simulink model "IEEE33_SmartInverter_Physical"  (R2026a)
settings: Solver=ode23t  StopTime=2.4  MaxStep=1e-3
PreLoadFcn:
  | try, startup_project(); addpath(fullfile(pwd,'simulink_physical')); if evalin('base','exist(''simscape_pv_p_commands'',''var'')') == 0, prepare_ieee33_simscape_inputs(80,'partial_cloud','hybrid'); end; catch ME, disp(['Physical-model preload warning: ' ME.message]); end
undefined symbols (not defined in the file or in its folder): simscape_pv_capacity_kW
libraries: ee_lib x116, nesl_utility x111, fl_lib x34
(part 2 of 2)

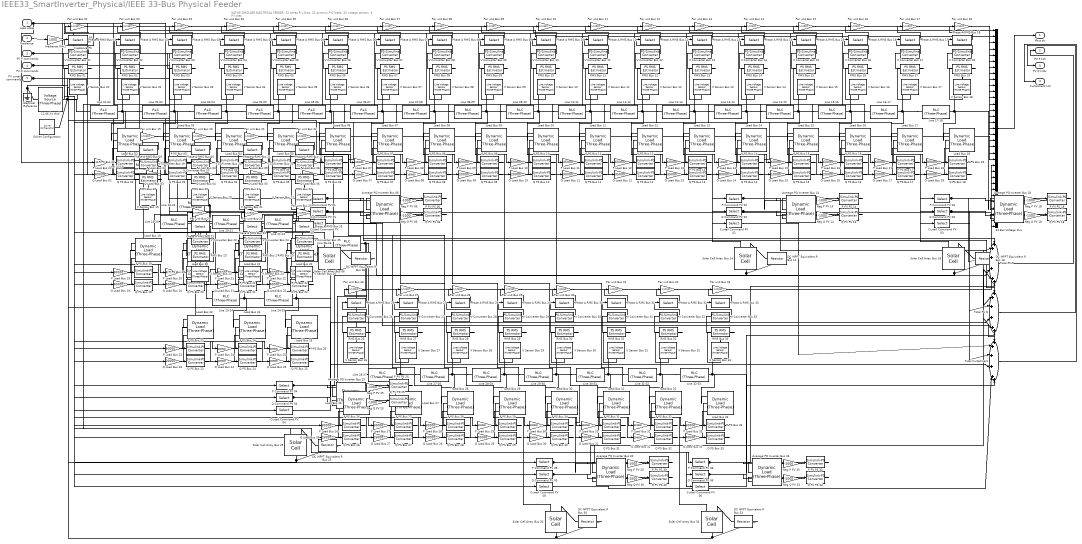
== system IEEE33_SmartInverter_Physical/IEEE 33-Bus Physical Feeder ==
  note: NATIVE SIMSCAPE ELECTRICAL FEEDER: 32 series R-L lines, 32 dynamic P-Q loads, 33 voltage sensors, 6 PV sites
  Load scale : Inport
  Irradiance : Inport  Port=2
  PV P commands : Inport  Port=3
  PV Q commands : Inport  Port=4
  PV curtail commands : Inport  Port=5
  12.66 kV Grid : ee_lib/Sources/Voltage Source (Three-Phase)  vline_rms=12660 V  shift=0 deg  freq=50 Hz  impedance_option=2  SShortCircuit=1e6 A*V  XR=15  R=0.001 Ohm  L=1e-6 H  harmonic_option=0  harmonic_orders=[5, 7, 11, 13]  harmonic_ratios=[.1, .1, .1, .1]  G_parasitic=0 1/Ohm  I_specify=off  I_priority=None  I=[0, 0, 0] A  I_nominal_specify=off  I_nominal_value=1  I_nominal_unit=A
  33 Bus Voltage Mux : Mux  Inputs=33
  Average PQ Inverter Bus 06 : ee_lib/Passive/Dynamic Load (Three-Phase)  port_option=ee.enum.threePhasePort.composite  FRated=50 Hz  Vline_rms_min=1000 V  tau=0.02 s  Vline_rms_ini=12660 V  Vang_ini=0 deg  gmin=1e-9 S
  Average PQ Inverter Bus {14,18,25,30,33} (5 alike) : ee_lib/Passive/Dynamic Load (Three-Phase)  port_option=ee.enum.threePhasePort.composite  FRated=50 Hz  Vline_rms_min=1000 V  tau=0.02 s  Vline_rms_ini=12660 V  Vang_ini=0 deg  gmin=1e-9 S
  Curtail Command PV 01 : Selector  InputPortWidth=6  IndexOptions=Index vector (dialog)  Indices=1  OutputSizes=1
  Curtail Command PV 02 : Selector  InputPortWidth=6  IndexOptions=Index vector (dialog)  Indices=2  OutputSizes=1
  Curtail Command PV 03 : Selector  InputPortWidth=6  IndexOptions=Index vector (dialog)  Indices=3  OutputSizes=1
  Curtail Command PV 04 : Selector  InputPortWidth=6  IndexOptions=Index vector (dialog)  Indices=4  OutputSizes=1
  Curtail Command PV 05 : Selector  InputPortWidth=6  IndexOptions=Index vector (dialog)  Indices=5  OutputSizes=1
  Curtail Command PV 06 : Selector  InputPortWidth=6  IndexOptions=Index vector (dialog)  Indices=6  OutputSizes=1
  DC MPPT Equivalent R Bus 06 : ee_lib/Passive/Resistor  R=(0.8*0.6*600)^2/max(simscape_pv_capacity_kW(1)*1000,1) Ohm  enable_R_tol=ee.enum.toleranceApplication.none  R_tol=5  tol_distribution=ee.enum.toleranceDistribution.uniform  nSigma=4  enable_operating_limits=ee.enum.enable.no  operating_limit_action=ee.enum.passive.reportOpLim.warn  power_rating=1 W  max_working_voltage=100 V  noise_mode=ee.enum.sources.noise.Disabled  Tdevice=25 degC  sample_time=1e-3 s  repeatability=ee.enum.ic.repeatability.notRepeatable  user_seed=0  auto_seed=3499211588  power_derating_T1=70 degC  power_derating_T2=155 degC  operating_temperature_range_vec=[-50, 150] degC  alpha=3.93e-3 1/K  Tmeas=25 degC  thermal_mass=100 J/K  temperature_specify=off  temperature_priority=High  temperature=298.15 K  temperature_nominal_specify=off  temperature_nominal_value=1  temperature_nominal_unit=K
  DC MPPT Equivalent R Bus 14 : ee_lib/Passive/Resistor  R=(0.8*0.6*600)^2/max(simscape_pv_capacity_kW(2)*1000,1) Ohm  enable_R_tol=ee.enum.toleranceApplication.none  R_tol=5  tol_distribution=ee.enum.toleranceDistribution.uniform  nSigma=4  enable_operating_limits=ee.enum.enable.no  operating_limit_action=ee.enum.passive.reportOpLim.warn  power_rating=1 W  max_working_voltage=100 V  noise_mode=ee.enum.sources.noise.Disabled  Tdevice=25 degC  sample_time=1e-3 s  repeatability=ee.enum.ic.repeatability.notRepeatable  user_seed=0  auto_seed=3890346746  power_derating_T1=70 degC  power_derating_T2=155 degC  operating_temperature_range_vec=[-50, 150] degC  alpha=3.93e-3 1/K  Tmeas=25 degC  thermal_mass=100 J/K  temperature_specify=off  temperature_priority=High  temperature=298.15 K  temperature_nominal_specify=off  temperature_nominal_value=1  temperature_nominal_unit=K
  DC MPPT Equivalent R Bus 18 : ee_lib/Passive/Resistor  R=(0.8*0.6*600)^2/max(simscape_pv_capacity_kW(3)*1000,1) Ohm  enable_R_tol=ee.enum.toleranceApplication.none  R_tol=5  tol_distribution=ee.enum.toleranceDistribution.uniform  nSigma=4  enable_operating_limits=ee.enum.enable.no  operating_limit_action=ee.enum.passive.reportOpLim.warn  power_rating=1 W  max_working_voltage=100 V  noise_mode=ee.enum.sources.noise.Disabled  Tdevice=25 degC  sample_time=1e-3 s  repeatability=ee.enum.ic.repeatability.notRepeatable  user_seed=0  auto_seed=545404223  power_derating_T1=70 degC  power_derating_T2=155 degC  operating_temperature_range_vec=[-50, 150] degC  alpha=3.93e-3 1/K  Tmeas=25 degC  thermal_mass=100 J/K  temperature_specify=off  temperature_priority=High  temperature=298.15 K  temperature_nominal_specify=off  temperature_nominal_value=1  temperature_nominal_unit=K
  DC MPPT Equivalent R Bus 25 : ee_lib/Passive/Resistor  R=(0.8*0.6*600)^2/max(simscape_pv_capacity_kW(4)*1000,1) Ohm  enable_R_tol=ee.enum.toleranceApplication.none  R_tol=5  tol_distribution=ee.enum.toleranceDistribution.uniform  nSigma=4  enable_operating_limits=ee.enum.enable.no  operating_limit_action=ee.enum.passive.reportOpLim.warn  power_rating=1 W  max_working_voltage=100 V  noise_mode=ee.enum.sources.noise.Disabled  Tdevice=25 degC  sample_time=1e-3 s  repeatability=ee.enum.ic.repeatability.notRepeatable  user_seed=0  auto_seed=3922919431  power_derating_T1=70 degC  power_derating_T2=155 degC  operating_temperature_range_vec=[-50, 150] degC  alpha=3.93e-3 1/K  Tmeas=25 degC  thermal_mass=100 J/K  temperature_specify=off  temperature_priority=High  temperature=298.15 K  temperature_nominal_specify=off  temperature_nominal_value=1  temperature_nominal_unit=K
  DC MPPT Equivalent R Bus 30 : ee_lib/Passive/Resistor  R=(0.8*0.6*600)^2/max(simscape_pv_capacity_kW(5)*1000,1) Ohm  enable_R_tol=ee.enum.toleranceApplication.none  R_tol=5  tol_distribution=ee.enum.toleranceDistribution.uniform  nSigma=4  enable_operating_limits=ee.enum.enable.no  operating_limit_action=ee.enum.passive.reportOpLim.warn  power_rating=1 W  max_working_voltage=100 V  noise_mode=ee.enum.sources.noise.Disabled  Tdevice=25 degC  sample_time=1e-3 s  repeatability=ee.enum.ic.repeatability.notRepeatable  user_seed=0  auto_seed=2715962282  power_derating_T1=70 degC  power_derating_T2=155 degC  operating_temperature_range_vec=[-50, 150] degC  alpha=3.93e-3 1/K  Tmeas=25 degC  thermal_mass=100 J/K  temperature_specify=off  temperature_priority=High  temperature=298.15 K  temperature_nominal_specify=off  temperature_nominal_value=1  temperature_nominal_unit=K
  DC MPPT Equivalent R Bus 33 : ee_lib/Passive/Resistor  R=(0.8*0.6*600)^2/max(simscape_pv_capacity_kW(6)*1000,1) Ohm  enable_R_tol=ee.enum.toleranceApplication.none  R_tol=5  tol_distribution=ee.enum.toleranceDistribution.uniform  nSigma=4  enable_operating_limits=ee.enum.enable.no  operating_limit_action=ee.enum.passive.reportOpLim.warn  power_rating=1 W  max_working_voltage=100 V  noise_mode=ee.enum.sources.noise.Disabled  Tdevice=25 degC  sample_time=1e-3 s  repeatability=ee.enum.ic.repeatability.notRepeatable  user_seed=0  auto_seed=418932850  power_derating_T1=70 degC  power_derating_T2=155 degC  operating_temperature_range_vec=[-50, 150] degC  alpha=3.93e-3 1/K  Tmeas=25 degC  thermal_mass=100 J/K  temperature_specify=off  temperature_priority=High  temperature=298.15 K  temperature_nominal_specify=off  temperature_nominal_value=1  temperature_nominal_unit=K
  Electrical Reference : fl_lib/Electrical/Electrical Elements/Electrical Reference
  Irradiance PS : nesl_utility/Simulink-PS Converter  PhysicalDomain=network_engine_domain  SubClassName=ps_input  LeftPortType=input  RightPortType=output  PseudoPeriodic=off  Frequencies=[]  NoiseDistribution=none  NoiseParameters=[]  Unit=W/m^2  AffineConversion=off  FilteringAndDerivatives=provide  SimscapeFilterOrder=1  InputFilterTimeConstant=0.001  UdotUserProvided=0
  Irradiance Wm2 : Gain  Gain=1000
  Line 01-02 : ee_lib/Passive/RLC Assemblies/RLC (Three-Phase)  port_option=ee.enum.threePhasePort.composite  component_structure=ee.enum.rlc.structure.SeriesRL  R=0.0922 Ohm  L=0.000149605646506 H  C=1e-6 F  R_parasitic=0 Ohm  G_parasitic=1e-9 1/Ohm  IL_specify=off  IL_priority=High  IL=[0, 0, 0] A  IL_nominal_specify=off  IL_nominal_value=1  IL_nominal_unit=A  VC_specify=off  VC_priority=High  VC=[0, 0, 0] V  VC_nominal_specify=off  VC_nominal_value=1  VC_nominal_unit=V
  Line 02-03 : ee_lib/Passive/RLC Assemblies/RLC (Three-Phase)  port_option=ee.enum.threePhasePort.composite  component_structure=ee.enum.rlc.structure.SeriesRL  R=0.493 Ohm  L=0.000799276124207 H  C=1e-6 F  R_parasitic=0 Ohm  G_parasitic=1e-9 1/Ohm  IL_specify=off  IL_priority=High  IL=[0, 0, 0] A  IL_nominal_specify=off  IL_nominal_value=1  IL_nominal_unit=A  VC_specify=off  VC_priority=High  VC=[0, 0, 0] V  VC_nominal_specify=off  VC_nominal_value=1  VC_nominal_unit=V
  Line 02-19 : ee_lib/Passive/RLC Assemblies/RLC (Three-Phase)  port_option=ee.enum.threePhasePort.composite  component_structure=ee.enum.rlc.structure.SeriesRL  R=0.164 Ohm  L=0.000498154971878 H  C=1e-6 F  R_parasitic=0 Ohm  G_parasitic=1e-9 1/Ohm  IL_specify=off  IL_priority=High  IL=[0, 0, 0] A  IL_nominal_specify=off  IL_nominal_value=1  IL_nominal_unit=A  VC_specify=off  VC_priority=High  VC=[0, 0, 0] V  VC_nominal_specify=off  VC_nominal_value=1  VC_nominal_unit=V
  Line 03-04 : ee_lib/Passive/RLC Assemblies/RLC (Three-Phase)  port_option=ee.enum.threePhasePort.composite  component_structure=ee.enum.rlc.structure.SeriesRL  R=0.366 Ohm  L=0.000593329627847 H  C=1e-6 F  R_parasitic=0 Ohm  G_parasitic=1e-9 1/Ohm  IL_specify=off  IL_priority=High  IL=[0, 0, 0] A  IL_nominal_specify=off  IL_nominal_value=1  IL_nominal_unit=A  VC_specify=off  VC_priority=High  VC=[0, 0, 0] V  VC_nominal_specify=off  VC_nominal_value=1  VC_nominal_unit=V
  Line 03-23 : ee_lib/Passive/RLC Assemblies/RLC (Three-Phase)  port_option=ee.enum.threePhasePort.composite  component_structure=ee.enum.rlc.structure.SeriesRL  R=0.4512 Ohm  L=0.000981349379105 H  C=1e-6 F  R_parasitic=0 Ohm  G_parasitic=1e-9 1/Ohm  IL_specify=off  IL_priority=High  IL=[0, 0, 0] A  IL_nominal_specify=off  IL_nominal_value=1  IL_nominal_unit=A  VC_specify=off  VC_priority=High  VC=[0, 0, 0] V  VC_nominal_specify=off  VC_nominal_value=1  VC_nominal_unit=V
  Line 04-05 : ee_lib/Passive/RLC Assemblies/RLC (Three-Phase)  port_option=ee.enum.threePhasePort.composite  component_structure=ee.enum.rlc.structure.SeriesRL  R=0.3811 Ohm  L=0.000617839489083 H  C=1e-6 F  R_parasitic=0 Ohm  G_parasitic=1e-9 1/Ohm  IL_specify=off  IL_priority=High  IL=[0, 0, 0] A  IL_nominal_specify=off  IL_nominal_value=1  IL_nominal_unit=A  VC_specify=off  VC_priority=High  VC=[0, 0, 0] V  VC_nominal_specify=off  VC_nominal_value=1  VC_nominal_unit=V
  Line 05-06 : ee_lib/Passive/RLC Assemblies/RLC (Three-Phase)  port_option=ee.enum.threePhasePort.composite  component_structure=ee.enum.rlc.structure.SeriesRL  R=0.819 Ohm  L=0.00225045089532 H  C=1e-6 F  R_parasitic=0 Ohm  G_parasitic=1e-9 1/Ohm  IL_specify=off  IL_priority=High  IL=[0, 0, 0] A  IL_nominal_specify=off  IL_nominal_value=1  IL_nominal_unit=A  VC_specify=off  VC_priority=High  VC=[0, 0, 0] V  VC_nominal_specify=off  VC_nominal_value=1  VC_nominal_unit=V
  Line 06-07 : ee_lib/Passive/RLC Assemblies/RLC (Three-Phase)  port_option=ee.enum.threePhasePort.composite  component_structure=ee.enum.rlc.structure.SeriesRL  R=0.1872 Ohm  L=0.00196970157571 H  C=1e-6 F  R_parasitic=0 Ohm  G_parasitic=1e-9 1/Ohm  IL_specify=off  IL_priority=High  IL=[0, 0, 0] A  IL_nominal_specify=off  IL_nominal_value=1  IL_nominal_unit=A  VC_specify=off  VC_priority=High  VC=[0, 0, 0] V  VC_nominal_specify=off  VC_nominal_value=1  VC_nominal_unit=V
  Line 06-26 : ee_lib/Passive/RLC Assemblies/RLC (Three-Phase)  port_option=ee.enum.threePhasePort.composite  component_structure=ee.enum.rlc.structure.SeriesRL  R=0.203 Ohm  L=0.000329132422314 H  C=1e-6 F  R_parasitic=0 Ohm  G_parasitic=1e-9 1/Ohm  IL_specify=off  IL_priority=High  IL=[0, 0, 0] A  IL_nominal_specify=off  IL_nominal_value=1  IL_nominal_unit=A  VC_specify=off  VC_priority=High  VC=[0, 0, 0] V  VC_nominal_specify=off  VC_nominal_value=1  VC_nominal_unit=V
  Line 07-08 : ee_lib/Passive/RLC Assemblies/RLC (Three-Phase)  port_option=ee.enum.threePhasePort.composite  component_structure=ee.enum.rlc.structure.SeriesRL  R=1.7114 Ohm  L=0.00393144540426 H  C=1e-6 F  R_parasitic=0 Ohm  G_parasitic=1e-9 1/Ohm  IL_specify=off  IL_priority=High  IL=[0, 0, 0] A  IL_nominal_specify=off  IL_nominal_value=1  IL_nominal_unit=A  VC_specify=off  VC_priority=High  VC=[0, 0, 0] V  VC_nominal_specify=off  VC_nominal_value=1  VC_nominal_unit=V
  Line 08-09 : ee_lib/Passive/RLC Assemblies/RLC (Three-Phase)  port_option=ee.enum.threePhasePort.composite  component_structure=ee.enum.rlc.structure.SeriesRL  R=1.03 Ohm  L=0.00235549315776 H  C=1e-6 F  R_parasitic=0 Ohm  G_parasitic=1e-9 1/Ohm  IL_specify=off  IL_priority=High  IL=[0, 0, 0] A  IL_nominal_specify=off  IL_nominal_value=1  IL_nominal_unit=A  VC_specify=off  VC_priority=High  VC=[0, 0, 0] V  VC_nominal_specify=off  VC_nominal_value=1  VC_nominal_unit=V
  Line 09-10 : ee_lib/Passive/RLC Assemblies/RLC (Three-Phase)  port_option=ee.enum.threePhasePort.composite  component_structure=ee.enum.rlc.structure.SeriesRL  R=1.044 Ohm  L=0.00235549315776 H  C=1e-6 F  R_parasitic=0 Ohm  G_parasitic=1e-9 1/Ohm  IL_specify=off  IL_priority=High  IL=[0, 0, 0] A  IL_nominal_specify=off  IL_nominal_value=1  IL_nominal_unit=A  VC_specify=off  VC_priority=High  VC=[0, 0, 0] V  VC_nominal_specify=off  VC_nominal_value=1  VC_nominal_unit=V
  Line 10-11 : ee_lib/Passive/RLC Assemblies/RLC (Three-Phase)  port_option=ee.enum.threePhasePort.composite  component_structure=ee.enum.rlc.structure.SeriesRL  R=0.1966 Ohm  L=0.000206901426019 H  C=1e-6 F  R_parasitic=0 Ohm  G_parasitic=1e-9 1/Ohm  IL_specify=off  IL_priority=High  IL=[0, 0, 0] A  IL_nominal_specify=off  IL_nominal_value=1  IL_nominal_unit=A  VC_specify=off  VC_priority=High  VC=[0, 0, 0] V  VC_nominal_specify=off  VC_nominal_value=1  VC_nominal_unit=V
  Line 11-12 : ee_lib/Passive/RLC Assemblies/RLC (Three-Phase)  port_option=ee.enum.threePhasePort.composite  component_structure=ee.enum.rlc.structure.SeriesRL  R=0.3744 Ohm  L=0.000394067639096 H  C=1e-6 F  R_parasitic=0 Ohm  G_parasitic=1e-9 1/Ohm  IL_specify=off  IL_priority=High  IL=[0, 0, 0] A  IL_nominal_specify=off  IL_nominal_value=1  IL_nominal_unit=A  VC_specify=off  VC_priority=High  VC=[0, 0, 0] V  VC_nominal_specify=off  VC_nominal_value=1  VC_nominal_unit=V
  Line 12-13 : ee_lib/Passive/RLC Assemblies/RLC (Three-Phase)  port_option=ee.enum.threePhasePort.composite  component_structure=ee.enum.rlc.structure.SeriesRL  R=1.468 Ohm  L=0.00367647918542 H  C=1e-6 F  R_parasitic=0 Ohm  G_parasitic=1e-9 1/Ohm  IL_specify=off  IL_priority=High  IL=[0, 0, 0] A  IL_nominal_specify=off  IL_nominal_value=1  IL_nominal_unit=A  VC_specify=off  VC_priority=High  VC=[0, 0, 0] V  VC_nominal_specify=off  VC_nominal_value=1  VC_nominal_unit=V
  Line 13-14 : ee_lib/Passive/RLC Assemblies/RLC (Three-Phase)  port_option=ee.enum.threePhasePort.composite  component_structure=ee.enum.rlc.structure.SeriesRL  R=0.5416 Ohm  L=0.0022692311786 H  C=1e-6 F  R_parasitic=0 Ohm  G_parasitic=1e-9 1/Ohm  IL_specify=off  IL_priority=High  IL=[0, 0, 0] A  IL_nominal_specify=off  IL_nominal_value=1  IL_nominal_unit=A  VC_specify=off  VC_priority=High  VC=[0, 0, 0] V  VC_nominal_specify=off  VC_nominal_value=1  VC_nominal_unit=V
  Line 14-15 : ee_lib/Passive/RLC Assemblies/RLC (Three-Phase)  port_option=ee.enum.threePhasePort.composite  component_structure=ee.enum.rlc.structure.SeriesRL  R=0.591 Ohm  L=0.00167431000133 H  C=1e-6 F  R_parasitic=0 Ohm  G_parasitic=1e-9 1/Ohm  IL_specify=off  IL_priority=High  IL=[0, 0, 0] A  IL_nominal_specify=off  IL_nominal_value=1  IL_nominal_unit=A  VC_specify=off  VC_priority=High  VC=[0, 0, 0] V  VC_nominal_specify=off  VC_nominal_value=1  VC_nominal_unit=V
  Line 15-16 : ee_lib/Passive/RLC Assemblies/RLC (Three-Phase)  port_option=ee.enum.threePhasePort.composite  component_structure=ee.enum.rlc.structure.SeriesRL  R=0.7463 Ohm  L=0.0017347888797 H  C=1e-6 F  R_parasitic=0 Ohm  G_parasitic=1e-9 1/Ohm  IL_specify=off  IL_priority=High  IL=[0, 0, 0] A  IL_nominal_specify=off  IL_nominal_value=1  IL_nominal_unit=A  VC_specify=off  VC_priority=High  VC=[0, 0, 0] V  VC_nominal_specify=off  VC_nominal_value=1  VC_nominal_unit=V
  Line 16-17 : ee_lib/Passive/RLC Assemblies/RLC (Three-Phase)  port_option=ee.enum.threePhasePort.composite  component_structure=ee.enum.rlc.structure.SeriesRL  R=1.289 Ohm  L=0.00547811314122 H  C=1e-6 F  R_parasitic=0 Ohm  G_parasitic=1e-9 1/Ohm  IL_specify=off  IL_priority=High  IL=[0, 0, 0] A  IL_nominal_specify=off  IL_nominal_value=1  IL_nominal_unit=A  VC_specify=off  VC_priority=High  VC=[0, 0, 0] V  VC_nominal_specify=off  VC_nominal_value=1  VC_nominal_unit=V
  Line 17-18 : ee_lib/Passive/RLC Assemblies/RLC (Three-Phase)  port_option=ee.enum.threePhasePort.composite  component_structure=ee.enum.rlc.structure.SeriesRL  R=0.732 Ohm  L=0.00182709874669 H  C=1e-6 F  R_parasitic=0 Ohm  G_parasitic=1e-9 1/Ohm  IL_specify=off  IL_priority=High  IL=[0, 0, 0] A  IL_nominal_specify=off  IL_nominal_value=1  IL_nominal_unit=A  VC_specify=off  VC_priority=High  VC=[0, 0, 0] V  VC_nominal_specify=off  VC_nominal_value=1  VC_nominal_unit=V
  Line 19-20 : ee_lib/Passive/RLC Assemblies/RLC (Three-Phase)  port_option=ee.enum.threePhasePort.composite  component_structure=ee.enum.rlc.structure.SeriesRL  R=1.5042 Ohm  L=0.00431437219734 H  C=1e-6 F  R_parasitic=0 Ohm  G_parasitic=1e-9 1/Ohm  IL_specify=off  IL_priority=High  IL=[0, 0, 0] A  IL_nominal_specify=off  IL_nominal_value=1  IL_nominal_unit=A  VC_specify=off  VC_priority=High  VC=[0, 0, 0] V  VC_nominal_specify=off  VC_nominal_value=1  VC_nominal_unit=V
  Line 20-21 : ee_lib/Passive/RLC Assemblies/RLC (Three-Phase)  port_option=ee.enum.threePhasePort.composite  component_structure=ee.enum.rlc.structure.SeriesRL  R=0.4095 Ohm  L=0.0015227944955 H  C=1e-6 F  R_parasitic=0 Ohm  G_parasitic=1e-9 1/Ohm  IL_specify=off  IL_priority=High  IL=[0, 0, 0] A  IL_nominal_specify=off  IL_nominal_value=1  IL_nominal_unit=A  VC_specify=off  VC_priority=High  VC=[0, 0, 0] V  VC_nominal_specify=off  VC_nominal_value=1  VC_nominal_unit=V
  Line 21-22 : ee_lib/Passive/RLC Assemblies/RLC (Three-Phase)  port_option=ee.enum.threePhasePort.composite  component_structure=ee.enum.rlc.structure.SeriesRL  R=0.7089 Ohm  L=0.0029835185632 H  C=1e-6 F  R_parasitic=0 Ohm  G_parasitic=1e-9 1/Ohm  IL_specify=off  IL_priority=High  IL=[0, 0, 0] A  IL_nominal_specify=off  IL_nominal_value=1  IL_nominal_unit=A  VC_specify=off  VC_priority=High  VC=[0, 0, 0] V  VC_nominal_specify=off  VC_nominal_value=1  VC_nominal_unit=V
  Line 23-24 : ee_lib/Passive/RLC Assemblies/RLC (Three-Phase)  port_option=ee.enum.threePhasePort.composite  component_structure=ee.enum.rlc.structure.SeriesRL  R=0.898 Ohm  L=0.00225713540293 H  C=1e-6 F  R_parasitic=0 Ohm  G_parasitic=1e-9 1/Ohm  IL_specify=off  IL_priority=High  IL=[0, 0, 0] A  IL_nominal_specify=off  IL_nominal_value=1  IL_nominal_unit=A  VC_specify=off  VC_priority=High  VC=[0, 0, 0] V  VC_nominal_specify=off  VC_nominal_value=1  VC_nominal_unit=V
  Line 24-25 : ee_lib/Passive/RLC Assemblies/RLC (Three-Phase)  port_option=ee.enum.threePhasePort.composite  component_structure=ee.enum.rlc.structure.SeriesRL  R=0.896 Ohm  L=0.00223167061203 H  C=1e-6 F  R_parasitic=0 Ohm  G_parasitic=1e-9 1/Ohm  IL_specify=off  IL_priority=High  IL=[0, 0, 0] A  IL_nominal_specify=off  IL_nominal_value=1  IL_nominal_unit=A  VC_specify=off  VC_priority=High  VC=[0, 0, 0] V  VC_nominal_specify=off  VC_nominal_value=1  VC_nominal_unit=V
  Line 26-27 : ee_lib/Passive/RLC Assemblies/RLC (Three-Phase)  port_option=ee.enum.threePhasePort.composite  component_structure=ee.enum.rlc.structure.SeriesRL  R=0.2842 Ohm  L=0.000460594405308 H  C=1e-6 F  R_parasitic=0 Ohm  G_parasitic=1e-9 1/Ohm  IL_specify=off  IL_priority=High  IL=[0, 0, 0] A  IL_nominal_specify=off  IL_nominal_value=1  IL_nominal_unit=A  VC_specify=off  VC_priority=High  VC=[0, 0, 0] V  VC_nominal_specify=off  VC_nominal_value=1  VC_nominal_unit=V
  Line 27-28 : ee_lib/Passive/RLC Assemblies/RLC (Three-Phase)  port_option=ee.enum.threePhasePort.composite  component_structure=ee.enum.rlc.structure.SeriesRL  R=1.059 Ohm  L=0.0029720594073 H  C=1e-6 F  R_parasitic=0 Ohm  G_parasitic=1e-9 1/Ohm  IL_specify=off  IL_priority=High  IL=[0, 0, 0] A  IL_nominal_specify=off  IL_nominal_value=1  IL_nominal_unit=A  VC_specify=off  VC_priority=High  VC=[0, 0, 0] V  VC_nominal_specify=off  VC_nominal_value=1  VC_nominal_unit=V
  Line 28-29 : ee_lib/Passive/RLC Assemblies/RLC (Three-Phase)  port_option=ee.enum.threePhasePort.composite  component_structure=ee.enum.rlc.structure.SeriesRL  R=0.8042 Ohm  L=0.0022300790626 H  C=1e-6 F  R_parasitic=0 Ohm  G_parasitic=1e-9 1/Ohm  IL_specify=off  IL_priority=High  IL=[0, 0, 0] A  IL_nominal_specify=off  IL_nominal_value=1  IL_nominal_unit=A  VC_specify=off  VC_priority=High  VC=[0, 0, 0] V  VC_nominal_specify=off  VC_nominal_value=1  VC_nominal_unit=V
  Line 29-30 : ee_lib/Passive/RLC Assemblies/RLC (Three-Phase)  port_option=ee.enum.threePhasePort.composite  component_structure=ee.enum.rlc.structure.SeriesRL  R=0.5075 Ohm  L=0.000822831055785 H  C=1e-6 F  R_parasitic=0 Ohm  G_parasitic=1e-9 1/Ohm  IL_specify=off  IL_priority=High  IL=[0, 0, 0] A  IL_nominal_specify=off  IL_nominal_value=1  IL_nominal_unit=A  VC_specify=off  VC_priority=High  VC=[0, 0, 0] V  VC_nominal_specify=off  VC_nominal_value=1  VC_nominal_unit=V
  Line 30-31 : ee_lib/Passive/RLC Assemblies/RLC (Three-Phase)  port_option=ee.enum.threePhasePort.composite  component_structure=ee.enum.rlc.structure.SeriesRL  R=0.9744 Ohm  L=0.00306532420395 H  C=1e-6 F  R_parasitic=0 Ohm  G_parasitic=1e-9 1/Ohm  IL_specify=off  IL_priority=High  IL=[0, 0, 0] A  IL_nominal_specify=off  IL_nominal_value=1  IL_nominal_unit=A  VC_specify=off  VC_priority=High  VC=[0, 0, 0] V  VC_nominal_specify=off  VC_nominal_value=1  VC_nominal_unit=V
  Line 31-32 : ee_lib/Passive/RLC Assemblies/RLC (Three-Phase)  port_option=ee.enum.threePhasePort.composite  component_structure=ee.enum.rlc.structure.SeriesRL  R=0.3105 Ohm  L=0.0011519634781 H  C=1e-6 F  R_parasitic=0 Ohm  G_parasitic=1e-9 1/Ohm  IL_specify=off  IL_priority=High  IL=[0, 0, 0] A  IL_nominal_specify=off  IL_nominal_value=1  IL_nominal_unit=A  VC_specify=off  VC_priority=High  VC=[0, 0, 0] V  VC_nominal_specify=off  VC_nominal_value=1  VC_nominal_unit=V
  Line 32-33 : ee_lib/Passive/RLC Assemblies/RLC (Three-Phase)  port_option=ee.enum.threePhasePort.composite  component_structure=ee.enum.rlc.structure.SeriesRL  R=0.341 Ohm  L=0.00168767901655 H  C=1e-6 F  R_parasitic=0 Ohm  G_parasitic=1e-9 1/Ohm  IL_specify=off  IL_priority=High  IL=[0, 0, 0] A  IL_nominal_specify=off  IL_nominal_value=1  IL_nominal_unit=A  VC_specify=off  VC_priority=High  VC=[0, 0, 0] V  VC_nominal_specify=off  VC_nominal_value=1  VC_nominal_unit=V
  Load Bus 02 : ee_lib/Passive/Dynamic Load (Three-Phase)  port_option=ee.enum.threePhasePort.composite  FRated=50 Hz  Vline_rms_min=1000 V  tau=0.02 s  Vline_rms_ini=12660 V  Vang_ini=0 deg  gmin=1e-9 S
  Load Bus 03 : ee_lib/Passive/Dynamic Load (Three-Phase)  port_option=ee.enum.threePhasePort.composite  FRated=50 Hz  Vline_rms_min=1000 V  tau=0.02 s  Vline_rms_ini=12660 V  Vang_ini=0 deg  gmin=1e-9 S
  Load Bus 04 : ee_lib/Passive/Dynamic Load (Three-Phase)  port_option=ee.enum.threePhasePort.composite  FRated=50 Hz  Vline_rms_min=1000 V  tau=0.02 s  Vline_rms_ini=12660 V  Vang_ini=0 deg  gmin=1e-9 S
  Load Bus 05 : ee_lib/Passive/Dynamic Load (Three-Phase)  port_option=ee.enum.threePhasePort.composite  FRated=50 Hz  Vline_rms_min=1000 V  tau=0.02 s  Vline_rms_ini=12660 V  Vang_ini=0 deg  gmin=1e-9 S
  Load Bus 06 : ee_lib/Passive/Dynamic Load (Three-Phase)  port_option=ee.enum.threePhasePort.composite  FRated=50 Hz  Vline_rms_min=1000 V  tau=0.02 s  Vline_rms_ini=12660 V  Vang_ini=0 deg  gmin=1e-9 S
  Load Bus 07 : ee_lib/Passive/Dynamic Load (Three-Phase)  port_option=ee.enum.threePhasePort.composite  FRated=50 Hz  Vline_rms_min=1000 V  tau=0.02 s  Vline_rms_ini=12660 V  Vang_ini=0 deg  gmin=1e-9 S
  Load Bus 08 : ee_lib/Passive/Dynamic Load (Three-Phase)  port_option=ee.enum.threePhasePort.composite  FRated=50 Hz  Vline_rms_min=1000 V  tau=0.02 s  Vline_rms_ini=12660 V  Vang_ini=0 deg  gmin=1e-9 S
  Load Bus 09 : ee_lib/Passive/Dynamic Load (Three-Phase)  port_option=ee.enum.threePhasePort.composite  FRated=50 Hz  Vline_rms_min=1000 V  tau=0.02 s  Vline_rms_ini=12660 V  Vang_ini=0 deg  gmin=1e-9 S
  Load Bus {10..33} (24 alike) : ee_lib/Passive/Dynamic Load (Three-Phase)  port_option=ee.enum.threePhasePort.composite  FRated=50 Hz  Vline_rms_min=1000 V  tau=0.02 s  Vline_rms_ini=12660 V  Vang_ini=0 deg  gmin=1e-9 S
  Neg P PV 06 : Gain  Gain=-1000
  Neg P PV {14,18,25,30,33} (5 alike) : Gain  Gain=-1000
  Neg Q PV 06 : Gain  Gain=-1000
  Neg Q PV {14,18,25,30,33} (5 alike) : Gain  Gain=-1000
  P Command PV 01 : Selector  InputPortWidth=6  IndexOptions=Index vector (dialog)  Indices=1  OutputSizes=1
  P Command PV 02 : Selector  InputPortWidth=6  IndexOptions=Index vector (dialog)  Indices=2  OutputSizes=1
  P Command PV 03 : Selector  InputPortWidth=6  IndexOptions=Index vector (dialog)  Indices=3  OutputSizes=1
  P Command PV 04 : Selector  InputPortWidth=6  IndexOptions=Index vector (dialog)  Indices=4  OutputSizes=1
  P Command PV 05 : Selector  InputPortWidth=6  IndexOptions=Index vector (dialog)  Indices=5  OutputSizes=1
  P Command PV 06 : Selector  InputPortWidth=6  IndexOptions=Index vector (dialog)  Indices=6  OutputSizes=1
  P Load Bus 02 : Gain  Gain=100000
  P Load Bus 03 : Gain  Gain=90000
  P Load Bus 04 : Gain  Gain=120000
  P Load Bus 05 : Gain  Gain=60000
  P Load Bus 06 : Gain  Gain=60000
  P Load Bus 07 : Gain  Gain=200000
  P Load Bus 08 : Gain  Gain=200000
  P Load Bus 09 : Gain  Gain=60000
  P Load Bus {10,12..13,15..17,26..28,33} (10 alike) : Gain  Gain=60000
  P Load Bus 11 : Gain  Gain=45000
  P Load Bus 14 : Gain  Gain=120000
  P Load Bus {18..23} (6 alike) : Gain  Gain=90000
  P Load Bus 24 : Gain  Gain=420000
  P Load Bus 25 : Gain  Gain=420000
  P Load Bus 29 : Gain  Gain=120000
  P Load Bus 30 : Gain  Gain=200000
  P Load Bus 31 : Gain  Gain=150000
  P Load Bus 32 : Gain  Gain=210000
  P PS Bus 02 : nesl_utility/Simulink-PS Converter  PhysicalDomain=network_engine_domain  SubClassName=ps_input  LeftPortType=input  RightPortType=output  PseudoPeriodic=off  Frequencies=[]  NoiseDistribution=none  NoiseParameters=[]  Unit=W  AffineConversion=off  FilteringAndDerivatives=provide  SimscapeFilterOrder=1  InputFilterTimeConstant=0.001  UdotUserProvided=0
  P PS Bus 03 : nesl_utility/Simulink-PS Converter  PhysicalDomain=network_engine_domain  SubClassName=ps_input  LeftPortType=input  RightPortType=output  PseudoPeriodic=off  Frequencies=[]  NoiseDistribution=none  NoiseParameters=[]  Unit=W  AffineConversion=off  FilteringAndDerivatives=provide  SimscapeFilterOrder=1  InputFilterTimeConstant=0.001  UdotUserProvided=0
  P PS Bus 04 : nesl_utility/Simulink-PS Converter  PhysicalDomain=network_engine_domain  SubClassName=ps_input  LeftPortType=input  RightPortType=output  PseudoPeriodic=off  Frequencies=[]  NoiseDistribution=none  NoiseParameters=[]  Unit=W  AffineConversion=off  FilteringAndDerivatives=provide  SimscapeFilterOrder=1  InputFilterTimeConstant=0.001  UdotUserProvided=0
  P PS Bus 05 : nesl_utility/Simulink-PS Converter  PhysicalDomain=network_engine_domain  SubClassName=ps_input  LeftPortType=input  RightPortType=output  PseudoPeriodic=off  Frequencies=[]  NoiseDistribution=none  NoiseParameters=[]  Unit=W  AffineConversion=off  FilteringAndDerivatives=provide  SimscapeFilterOrder=1  InputFilterTimeConstant=0.001  UdotUserProvided=0
  P PS Bus 06 : nesl_utility/Simulink-PS Converter  PhysicalDomain=network_engine_domain  SubClassName=ps_input  LeftPortType=input  RightPortType=output  PseudoPeriodic=off  Frequencies=[]  NoiseDistribution=none  NoiseParameters=[]  Unit=W  AffineConversion=off  FilteringAndDerivatives=provide  SimscapeFilterOrder=1  InputFilterTimeConstant=0.001  UdotUserProvided=0
  P PS Bus 07 : nesl_utility/Simulink-PS Converter  PhysicalDomain=network_engine_domain  SubClassName=ps_input  LeftPortType=input  RightPortType=output  PseudoPeriodic=off  Frequencies=[]  NoiseDistribution=none  NoiseParameters=[]  Unit=W  AffineConversion=off  FilteringAndDerivatives=provide  SimscapeFilterOrder=1  InputFilterTimeConstant=0.001  UdotUserProvided=0
  P PS Bus 08 : nesl_utility/Simulink-PS Converter  PhysicalDomain=network_engine_domain  SubClassName=ps_input  LeftPortType=input  RightPortType=output  PseudoPeriodic=off  Frequencies=[]  NoiseDistribution=none  NoiseParameters=[]  Unit=W  AffineConversion=off  FilteringAndDerivatives=provide  SimscapeFilterOrder=1  InputFilterTimeConstant=0.001  UdotUserProvided=0
  P PS Bus 09 : nesl_utility/Simulink-PS Converter  PhysicalDomain=network_engine_domain  SubClassName=ps_input  LeftPortType=input  RightPortType=output  PseudoPeriodic=off  Frequencies=[]  NoiseDistribution=none  NoiseParameters=[]  Unit=W  AffineConversion=off  FilteringAndDerivatives=provide  SimscapeFilterOrder=1  InputFilterTimeConstant=0.001  UdotUserProvided=0
  P PS Bus {10..33} (24 alike) : nesl_utility/Simulink-PS Converter  PhysicalDomain=network_engine_domain  SubClassName=ps_input  LeftPortType=input  RightPortType=output  PseudoPeriodic=off  Frequencies=[]  NoiseDistribution=none  NoiseParameters=[]  Unit=W  AffineConversion=off  FilteringAndDerivatives=provide  SimscapeFilterOrder=1  InputFilterTimeConstant=0.001  UdotUserProvided=0
  P PV PS 06 : nesl_utility/Simulink-PS Converter  PhysicalDomain=network_engine_domain  SubClassName=ps_input  LeftPortType=input  RightPortType=output  PseudoPeriodic=off  Frequencies=[]  NoiseDistribution=none  NoiseParameters=[]  Unit=W  AffineConversion=off  FilteringAndDerivatives=provide  SimscapeFilterOrder=1  InputFilterTimeConstant=0.001  UdotUserProvided=0
  P PV PS {14,18,25,30,33} (5 alike) : nesl_utility/Simulink-PS Converter  PhysicalDomain=network_engine_domain  SubClassName=ps_input  LeftPortType=input  RightPortType=output  PseudoPeriodic=off  Frequencies=[]  NoiseDistribution=none  NoiseParameters=[]  Unit=W  AffineConversion=off  FilteringAndDerivatives=provide  SimscapeFilterOrder=1  InputFilterTimeConstant=0.001  UdotUserProvided=0
  Per unit Bus 01 : Gain  Gain=1/12660
  Per unit Bus 02 : Gain  Gain=1/12660
  Per unit Bus 03 : Gain  Gain=1/12660
  Per unit Bus 04 : Gain  Gain=1/12660
  Per unit Bus 05 : Gain  Gain=1/12660
  Per unit Bus 06 : Gain  Gain=1/12660
  Per unit Bus 07 : Gain  Gain=1/12660
  Per unit Bus 08 : Gain  Gain=1/12660
  Per unit Bus 09 : Gain  Gain=1/12660
  Per unit Bus {10..33} (24 alike) : Gain  Gain=1/12660
  Phase A RMS Bus 01 : Selector  InputPortWidth=3  IndexOptions=Index vector (dialog)  Indices=1  OutputSizes=1
  Phase A RMS Bus 02 : Selector  InputPortWidth=3  IndexOptions=Index vector (dialog)  Indices=1  OutputSizes=1
  Phase A RMS Bus 03 : Selector  InputPortWidth=3  IndexOptions=Index vector (dialog)  Indices=1  OutputSizes=1
  Phase A RMS Bus 04 : Selector  InputPortWidth=3  IndexOptions=Index vector (dialog)  Indices=1  OutputSizes=1
  Phase A RMS Bus 05 : Selector  InputPortWidth=3  IndexOptions=Index vector (dialog)  Indices=1  OutputSizes=1
  Phase A RMS Bus 06 : Selector  InputPortWidth=3  IndexOptions=Index vector (dialog)  Indices=1  OutputSizes=1
  Phase A RMS Bus 07 : Selector  InputPortWidth=3  IndexOptions=Index vector (dialog)  Indices=1  OutputSizes=1
  Phase A RMS Bus 08 : Selector  InputPortWidth=3  IndexOptions=Index vector (dialog)  Indices=1  OutputSizes=1
  Phase A RMS Bus 09 : Selector  InputPortWidth=3  IndexOptions=Index vector (dialog)  Indices=1  OutputSizes=1
  Phase A RMS Bus {10..33} (24 alike) : Selector  InputPortWidth=3  IndexOptions=Index vector (dialog)  Indices=1  OutputSizes=1
  Q Command PV 01 : Selector  InputPortWidth=6  IndexOptions=Index vector (dialog)  Indices=1  OutputSizes=1
  Q Command PV 02 : Selector  InputPortWidth=6  IndexOptions=Index vector (dialog)  Indices=2  OutputSizes=1
  Q Command PV 03 : Selector  InputPortWidth=6  IndexOptions=Index vector (dialog)  Indices=3  OutputSizes=1
  Q Command PV 04 : Selector  InputPortWidth=6  IndexOptions=Index vector (dialog)  Indices=4  OutputSizes=1
  Q Command PV 05 : Selector  InputPortWidth=6  IndexOptions=Index vector (dialog)  Indices=5  OutputSizes=1
  Q Command PV 06 : Selector  InputPortWidth=6  IndexOptions=Index vector (dialog)  Indices=6  OutputSizes=1
  Q Load Bus 02 : Gain  Gain=60000
  Q Load Bus 03 : Gain  Gain=40000
  Q Load Bus 04 : Gain  Gain=80000
  Q Load Bus 05 : Gain  Gain=30000
  Q Load Bus 06 : Gain  Gain=20000
  Q Load Bus 07 : Gain  Gain=100000
  Q Load Bus 08 : Gain  Gain=100000
  Q Load Bus 09 : Gain  Gain=20000
  Q Load Bus {10,16..17,28} (4 alike) : Gain  Gain=20000
  Q Load Bus 11 : Gain  Gain=30000
  Q Load Bus 12 : Gain  Gain=35000
  Q Load Bus 13 : Gain  Gain=35000
  Q Load Bus 14 : Gain  Gain=80000
  Q Load Bus 15 : Gain  Gain=10000
  Q Load Bus {18..22,33} (6 alike) : Gain  Gain=40000
  Q Load Bus 23 : Gain  Gain=50000
  Q Load Bus 24 : Gain  Gain=200000
  Q Load Bus 25 : Gain  Gain=200000
  Q Load Bus 26 : Gain  Gain=25000
  Q Load Bus 27 : Gain  Gain=25000
  Q Load Bus 29 : Gain  Gain=70000
  Q Load Bus 30 : Gain  Gain=600000
  Q Load Bus 31 : Gain  Gain=70000
  Q Load Bus 32 : Gain  Gain=100000
  Q PS Bus 02 : nesl_utility/Simulink-PS Converter  PhysicalDomain=network_engine_domain  SubClassName=ps_input  LeftPortType=input  RightPortType=output  PseudoPeriodic=off  Frequencies=[]  NoiseDistribution=none  NoiseParameters=[]  Unit=V*A  AffineConversion=off  FilteringAndDerivatives=provide  SimscapeFilterOrder=1  InputFilterTimeConstant=0.001  UdotUserProvided=0
  Q PS Bus 03 : nesl_utility/Simulink-PS Converter  PhysicalDomain=network_engine_domain  SubClassName=ps_input  LeftPortType=input  RightPortType=output  PseudoPeriodic=off  Frequencies=[]  NoiseDistribution=none  NoiseParameters=[]  Unit=V*A  AffineConversion=off  FilteringAndDerivatives=provide  SimscapeFilterOrder=1  InputFilterTimeConstant=0.001  UdotUserProvided=0
  Q PS Bus 04 : nesl_utility/Simulink-PS Converter  PhysicalDomain=network_engine_domain  SubClassName=ps_input  LeftPortType=input  RightPortType=output  PseudoPeriodic=off  Frequencies=[]  NoiseDistribution=none  NoiseParameters=[]  Unit=V*A  AffineConversion=off  FilteringAndDerivatives=provide  SimscapeFilterOrder=1  InputFilterTimeConstant=0.001  UdotUserProvided=0
  Q PS Bus 05 : nesl_utility/Simulink-PS Converter  PhysicalDomain=network_engine_domain  SubClassName=ps_input  LeftPortType=input  RightPortType=output  PseudoPeriodic=off  Frequencies=[]  NoiseDistribution=none  NoiseParameters=[]  Unit=V*A  AffineConversion=off  FilteringAndDerivatives=provide  SimscapeFilterOrder=1  InputFilterTimeConstant=0.001  UdotUserProvided=0
  Q PS Bus 06 : nesl_utility/Simulink-PS Converter  PhysicalDomain=network_engine_domain  SubClassName=ps_input  LeftPortType=input  RightPortType=output  PseudoPeriodic=off  Frequencies=[]  NoiseDistribution=none  NoiseParameters=[]  Unit=V*A  AffineConversion=off  FilteringAndDerivatives=provide  SimscapeFilterOrder=1  InputFilterTimeConstant=0.001  UdotUserProvided=0
  Q PS Bus 07 : nesl_utility/Simulink-PS Converter  PhysicalDomain=network_engine_domain  SubClassName=ps_input  LeftPortType=input  RightPortType=output  PseudoPeriodic=off  Frequencies=[]  NoiseDistribution=none  NoiseParameters=[]  Unit=V*A  AffineConversion=off  FilteringAndDerivatives=provide  SimscapeFilterOrder=1  InputFilterTimeConstant=0.001  UdotUserProvided=0
  Q PS Bus 08 : nesl_utility/Simulink-PS Converter  PhysicalDomain=network_engine_domain  SubClassName=ps_input  LeftPortType=input  RightPortType=output  PseudoPeriodic=off  Frequencies=[]  NoiseDistribution=none  NoiseParameters=[]  Unit=V*A  AffineConversion=off  FilteringAndDerivatives=provide  SimscapeFilterOrder=1  InputFilterTimeConstant=0.001  UdotUserProvided=0
  Q PS Bus 09 : nesl_utility/Simulink-PS Converter  PhysicalDomain=network_engine_domain  SubClassName=ps_input  LeftPortType=input  RightPortType=output  PseudoPeriodic=off  Frequencies=[]  NoiseDistribution=none  NoiseParameters=[]  Unit=V*A  AffineConversion=off  FilteringAndDerivatives=provide  SimscapeFilterOrder=1  InputFilterTimeConstant=0.001  UdotUserProvided=0
  Q PS Bus {10..33} (24 alike) : nesl_utility/Simulink-PS Converter  PhysicalDomain=network_engine_domain  SubClassName=ps_input  LeftPortType=input  RightPortType=output  PseudoPeriodic=off  Frequencies=[]  NoiseDistribution=none  NoiseParameters=[]  Unit=V*A  AffineConversion=off  FilteringAndDerivatives=provide  SimscapeFilterOrder=1  InputFilterTimeConstant=0.001  UdotUserProvided=0
  Q PV PS 06 : nesl_utility/Simulink-PS Converter  PhysicalDomain=network_engine_domain  SubClassName=ps_input  LeftPortType=input  RightPortType=output  PseudoPeriodic=off  Frequencies=[]  NoiseDistribution=none  NoiseParameters=[]  Unit=V*A  AffineConversion=off  FilteringAndDerivatives=provide  SimscapeFilterOrder=1  InputFilterTimeConstant=0.001  UdotUserProvided=0
  Q PV PS {14,18,25,30,33} (5 alike) : nesl_utility/Simulink-PS Converter  PhysicalDomain=network_engine_domain  SubClassName=ps_input  LeftPortType=input  RightPortType=output  PseudoPeriodic=off  Frequencies=[]  NoiseDistribution=none  NoiseParameters=[]  Unit=V*A  AffineConversion=off  FilteringAndDerivatives=provide  SimscapeFilterOrder=1  InputFilterTimeConstant=0.001  UdotUserProvided=0
  RMS Bus 01 : fl_lib/Physical Signals/Periodic Operators/PS RMS Estimator  f0=50 Hz
  RMS Bus 02 : fl_lib/Physical Signals/Periodic Operators/PS RMS Estimator  f0=50 Hz
  RMS Bus 03 : fl_lib/Physical Signals/Periodic Operators/PS RMS Estimator  f0=50 Hz
  RMS Bus 04 : fl_lib/Physical Signals/Periodic Operators/PS RMS Estimator  f0=50 Hz
  RMS Bus 05 : fl_lib/Physical Signals/Periodic Operators/PS RMS Estimator  f0=50 Hz
  RMS Bus 06 : fl_lib/Physical Signals/Periodic Operators/PS RMS Estimator  f0=50 Hz
  RMS Bus 07 : fl_lib/Physical Signals/Periodic Operators/PS RMS Estimator  f0=50 Hz
  RMS Bus 08 : fl_lib/Physical Signals/Periodic Operators/PS RMS Estimator  f0=50 Hz
  RMS Bus 09 : fl_lib/Physical Signals/Periodic Operators/PS RMS Estimator  f0=50 Hz
  RMS Bus {10..33} (24 alike) : fl_lib/Physical Signals/Periodic Operators/PS RMS Estimator  f0=50 Hz
  Solar Cell Array Bus 06 : ee_lib/Sources/Solar Cell  prm=ee.enum.sources.solar_cell_prm.datasheet  Isc=7.34 A  Voc=0.6 V  Is=1e-6 A  Is2=0 A  Iph=7.34 A  Ir0=1000 W/m^2  ec=1.5  N2=2  Rs=0 Ohm  Rp=inf Ohm  N_series=600  N_parallel=max(1,round(simscape_pv_capacity_kW(1)/2.1))  TIPH1=0 1/K  EG=1.11 eV  TXIS1=3  TXIS2=3  TRS1=0  TRP1=0  Tmeas=25 degC  TFIXED=25 degC  thermal_mass=100 J/K  initial_temperature=25 degC
  Solar Cell Array Bus 14 : ee_lib/Sources/Solar Cell  prm=ee.enum.sources.solar_cell_prm.datasheet  Isc=7.34 A  Voc=0.6 V  Is=1e-6 A  Is2=0 A  Iph=7.34 A  Ir0=1000 W/m^2  ec=1.5  N2=2  Rs=0 Ohm  Rp=inf Ohm  N_series=600  N_parallel=max(1,round(simscape_pv_capacity_kW(2)/2.1))  TIPH1=0 1/K  EG=1.11 eV  TXIS1=3  TXIS2=3  TRS1=0  TRP1=0  Tmeas=25 degC  TFIXED=25 degC  thermal_mass=100 J/K  initial_temperature=25 degC
  Solar Cell Array Bus 18 : ee_lib/Sources/Solar Cell  prm=ee.enum.sources.solar_cell_prm.datasheet  Isc=7.34 A  Voc=0.6 V  Is=1e-6 A  Is2=0 A  Iph=7.34 A  Ir0=1000 W/m^2  ec=1.5  N2=2  Rs=0 Ohm  Rp=inf Ohm  N_series=600  N_parallel=max(1,round(simscape_pv_capacity_kW(3)/2.1))  TIPH1=0 1/K  EG=1.11 eV  TXIS1=3  TXIS2=3  TRS1=0  TRP1=0  Tmeas=25 degC  TFIXED=25 degC  thermal_mass=100 J/K  initial_temperature=25 degC
  Solar Cell Array Bus 25 : ee_lib/Sources/Solar Cell  prm=ee.enum.sources.solar_cell_prm.datasheet  Isc=7.34 A  Voc=0.6 V  Is=1e-6 A  Is2=0 A  Iph=7.34 A  Ir0=1000 W/m^2  ec=1.5  N2=2  Rs=0 Ohm  Rp=inf Ohm  N_series=600  N_parallel=max(1,round(simscape_pv_capacity_kW(4)/2.1))  TIPH1=0 1/K  EG=1.11 eV  TXIS1=3  TXIS2=3  TRS1=0  TRP1=0  Tmeas=25 degC  TFIXED=25 degC  thermal_mass=100 J/K  initial_temperature=25 degC
  Solar Cell Array Bus 30 : ee_lib/Sources/Solar Cell  prm=ee.enum.sources.solar_cell_prm.datasheet  Isc=7.34 A  Voc=0.6 V  Is=1e-6 A  Is2=0 A  Iph=7.34 A  Ir0=1000 W/m^2  ec=1.5  N2=2  Rs=0 Ohm  Rp=inf Ohm  N_series=600  N_parallel=max(1,round(simscape_pv_capacity_kW(5)/2.1))  TIPH1=0 1/K  EG=1.11 eV  TXIS1=3  TXIS2=3  TRS1=0  TRP1=0  Tmeas=25 degC  TFIXED=25 degC  thermal_mass=100 J/K  initial_temperature=25 degC
  Solar Cell Array Bus 33 : ee_lib/Sources/Solar Cell  prm=ee.enum.sources.solar_cell_prm.datasheet  Isc=7.34 A  Voc=0.6 V  Is=1e-6 A  Is2=0 A  Iph=7.34 A  Ir0=1000 W/m^2  ec=1.5  N2=2  Rs=0 Ohm  Rp=inf Ohm  N_series=600  N_parallel=max(1,round(simscape_pv_capacity_kW(6)/2.1))  TIPH1=0 1/K  EG=1.11 eV  TXIS1=3  TXIS2=3  TRS1=0  TRP1=0  Tmeas=25 degC  TFIXED=25 degC  thermal_mass=100 J/K  initial_temperature=25 degC
  Solver Configuration : nesl_utility/Solver Configuration  PhysicalDomain=network_engine_domain  SubClassName=solver  LeftPortType=input  RightPortType=generic  Tones=[]  Harmonics=[]  SimulateNoise=off  Profile=off  UseLocalSampling=off  EnableSwitchedLinearOptims=on  FrequencyDomain=off  UseCCode=off  RelTol=0.001  AbsTol=0.001  MinStep=1e-09  ToWorkspace=off  RevertToSquareIcSolve=off  NumHomotopyIterations=100  PhasorMode=off  PhasorModeNumHarmonics=1  ConsistencySolver=NEWTON_XTOL_AFTER_FTOL  CanonicalOrdering=CANONICAL  OptimizeIntermediates=OPTIMIZED  IndexReductionMethod=DerivativeReplacement  DoDC=off  ResidualTolerance=1e-09  ConsistencyTolSource=GLOBAL  ConsistencyAbsTol=0.001  ConsistencyRelTol=0.001  ConsistencyTolFactor=0.001  UseLocalSolver=off  LocalSolverChoice=NE_BACKWARD_EULER_ADVANCER  ResolveIndetEquations=on  FunctionEvalNumThread=1  LocalSolverSampleTime=0.001  DoFixedCost=off  MaxNonlinIter=3  MaxModeIter=2  ComputeImpulses=off  ImpulseIterations=2  LinearAlgebra=auto  LinearAlgebraNumThread=0  EquationFormulation=NE_TIME_EF  DelaysMemoryBudget=1024  AutomaticFiltering=on  FilteringTimeConstant=0.001  PartitionStorageMethod=AS_NEEDED  PartitionMemoryBudget=1024  PartitionMethod=ROBUST  MultibodyUseLocalSolver=off  MultibodyLocalSolverChoice=ODE1  MultibodyLocalSolverSampleTime=0.001
  Total Curtailment : Sum  Inputs=++++++
  Total PV P : Sum  Inputs=++++++
  Total PV Q : Sum  Inputs=++++++
  V Converter Bus 01 : nesl_utility/PS-Simulink Converter  PhysicalDomain=network_engine_domain  SubClassName=ps_output  LeftPortType=input  RightPortType=output  PseudoPeriodic=off  Frequencies=[]  VectorFormat=inherit  Unit=V  AffineConversion=off
  V Converter Bus 02 : nesl_utility/PS-Simulink Converter  PhysicalDomain=network_engine_domain  SubClassName=ps_output  LeftPortType=input  RightPortType=output  PseudoPeriodic=off  Frequencies=[]  VectorFormat=inherit  Unit=V  AffineConversion=off
  V Converter Bus 03 : nesl_utility/PS-Simulink Converter  PhysicalDomain=network_engine_domain  SubClassName=ps_output  LeftPortType=input  RightPortType=output  PseudoPeriodic=off  Frequencies=[]  VectorFormat=inherit  Unit=V  AffineConversion=off
  V Converter Bus 04 : nesl_utility/PS-Simulink Converter  PhysicalDomain=network_engine_domain  SubClassName=ps_output  LeftPortType=input  RightPortType=output  PseudoPeriodic=off  Frequencies=[]  VectorFormat=inherit  Unit=V  AffineConversion=off
  V Converter Bus 05 : nesl_utility/PS-Simulink Converter  PhysicalDomain=network_engine_domain  SubClassName=ps_output  LeftPortType=input  RightPortType=output  PseudoPeriodic=off  Frequencies=[]  VectorFormat=inherit  Unit=V  AffineConversion=off
  V Converter Bus 06 : nesl_utility/PS-Simulink Converter  PhysicalDomain=network_engine_domain  SubClassName=ps_output  LeftPortType=input  RightPortType=output  PseudoPeriodic=off  Frequencies=[]  VectorFormat=inherit  Unit=V  AffineConversion=off
  V Converter Bus 07 : nesl_utility/PS-Simulink Converter  PhysicalDomain=network_engine_domain  SubClassName=ps_output  LeftPortType=input  RightPortType=output  PseudoPeriodic=off  Frequencies=[]  VectorFormat=inherit  Unit=V  AffineConversion=off
  V Converter Bus 08 : nesl_utility/PS-Simulink Converter  PhysicalDomain=network_engine_domain  SubClassName=ps_output  LeftPortType=input  RightPortType=output  PseudoPeriodic=off  Frequencies=[]  VectorFormat=inherit  Unit=V  AffineConversion=off
  V Converter Bus 09 : nesl_utility/PS-Simulink Converter  PhysicalDomain=network_engine_domain  SubClassName=ps_output  LeftPortType=input  RightPortType=output  PseudoPeriodic=off  Frequencies=[]  VectorFormat=inherit  Unit=V  AffineConversion=off
  V Converter Bus {10..33} (24 alike) : nesl_utility/PS-Simulink Converter  PhysicalDomain=network_engine_domain  SubClassName=ps_output  LeftPortType=input  RightPortType=output  PseudoPeriodic=off  Frequencies=[]  VectorFormat=inherit  Unit=V  AffineConversion=off
  V Sensor Bus 01 : ee_lib/Sensors & Transducers/Line Voltage Sensor (Three-Phase)  port_option=ee.enum.threePhasePort.composite
  V Sensor Bus 02 : ee_lib/Sensors & Transducers/Line Voltage Sensor (Three-Phase)  port_option=ee.enum.threePhasePort.composite
  V Sensor Bus 03 : ee_lib/Sensors & Transducers/Line Voltage Sensor (Three-Phase)  port_option=ee.enum.threePhasePort.composite
  V Sensor Bus 04 : ee_lib/Sensors & Transducers/Line Voltage Sensor (Three-Phase)  port_option=ee.enum.threePhasePort.composite
  V Sensor Bus 05 : ee_lib/Sensors & Transducers/Line Voltage Sensor (Three-Phase)  port_option=ee.enum.threePhasePort.composite
  V Sensor Bus 06 : ee_lib/Sensors & Transducers/Line Voltage Sensor (Three-Phase)  port_option=ee.enum.threePhasePort.composite
  V Sensor Bus 07 : ee_lib/Sensors & Transducers/Line Voltage Sensor (Three-Phase)  port_option=ee.enum.threePhasePort.composite
  V Sensor Bus 08 : ee_lib/Sensors & Transducers/Line Voltage Sensor (Three-Phase)  port_option=ee.enum.threePhasePort.composite
  V Sensor Bus 09 : ee_lib/Sensors & Transducers/Line Voltage Sensor (Three-Phase)  port_option=ee.enum.threePhasePort.composite
  V Sensor Bus {10..33} (24 alike) : ee_lib/Sensors & Transducers/Line Voltage Sensor (Three-Phase)  port_option=ee.enum.threePhasePort.composite
  Vbus pu : Outport
  PV P kW : Outport  Port=2
  PV Q kVAr : Outport  Port=3
  Curtailment kW : Outport  Port=4
  wires:
  V Converter Bus 01/1 -> Phase A RMS Bus 01/1
  Phase A RMS Bus 01/1 -> Per unit Bus 01/1
  Per unit Bus 01/1 -> 33 Bus Voltage Mux/1
  V Converter Bus 02/1 -> Phase A RMS Bus 02/1
  Phase A RMS Bus 02/1 -> Per unit Bus 02/1
  Per unit Bus 02/1 -> 33 Bus Voltage Mux/2
  V Converter Bus 03/1 -> Phase A RMS Bus 03/1
  Phase A RMS Bus 03/1 -> Per unit Bus 03/1
  Per unit Bus 03/1 -> 33 Bus Voltage Mux/3
  V Converter Bus 04/1 -> Phase A RMS Bus 04/1
  Phase A RMS Bus 04/1 -> Per unit Bus 04/1
  Per unit Bus 04/1 -> 33 Bus Voltage Mux/4
  V Converter Bus 05/1 -> Phase A RMS Bus 05/1
  Phase A RMS Bus 05/1 -> Per unit Bus 05/1
  Per unit Bus 05/1 -> 33 Bus Voltage Mux/5
  V Converter Bus 06/1 -> Phase A RMS Bus 06/1
  Phase A RMS Bus 06/1 -> Per unit Bus 06/1
  Per unit Bus 06/1 -> 33 Bus Voltage Mux/6
  V Converter Bus 07/1 -> Phase A RMS Bus 07/1
  Phase A RMS Bus 07/1 -> Per unit Bus 07/1
  Per unit Bus 07/1 -> 33 Bus Voltage Mux/7
  V Converter Bus 08/1 -> Phase A RMS Bus 08/1
  Phase A RMS Bus 08/1 -> Per unit Bus 08/1
  Per unit Bus 08/1 -> 33 Bus Voltage Mux/8
  V Converter Bus 09/1 -> Phase A RMS Bus 09/1
  Phase A RMS Bus 09/1 -> Per unit Bus 09/1
  Per unit Bus 09/1 -> 33 Bus Voltage Mux/9
  V Converter Bus 10/1 -> Phase A RMS Bus 10/1
  Phase A RMS Bus 10/1 -> Per unit Bus 10/1
  Per unit Bus 10/1 -> 33 Bus Voltage Mux/10
  V Converter Bus 11/1 -> Phase A RMS Bus 11/1
  Phase A RMS Bus 11/1 -> Per unit Bus 11/1
  Per unit Bus 11/1 -> 33 Bus Voltage Mux/11
  V Converter Bus 12/1 -> Phase A RMS Bus 12/1
  Phase A RMS Bus 12/1 -> Per unit Bus 12/1
  Per unit Bus 12/1 -> 33 Bus Voltage Mux/12
  V Converter Bus 13/1 -> Phase A RMS Bus 13/1
  Phase A RMS Bus 13/1 -> Per unit Bus 13/1
  Per unit Bus 13/1 -> 33 Bus Voltage Mux/13
  V Converter Bus 14/1 -> Phase A RMS Bus 14/1
  Phase A RMS Bus 14/1 -> Per unit Bus 14/1
  Per unit Bus 14/1 -> 33 Bus Voltage Mux/14
  V Converter Bus 15/1 -> Phase A RMS Bus 15/1
  Phase A RMS Bus 15/1 -> Per unit Bus 15/1
  Per unit Bus 15/1 -> 33 Bus Voltage Mux/15
  V Converter Bus 16/1 -> Phase A RMS Bus 16/1
  Phase A RMS Bus 16/1 -> Per unit Bus 16/1
  Per unit Bus 16/1 -> 33 Bus Voltage Mux/16
  V Converter Bus 17/1 -> Phase A RMS Bus 17/1
  Phase A RMS Bus 17/1 -> Per unit Bus 17/1
  Per unit Bus 17/1 -> 33 Bus Voltage Mux/17
  V Converter Bus 18/1 -> Phase A RMS Bus 18/1
  Phase A RMS Bus 18/1 -> Per unit Bus 18/1
  Per unit Bus 18/1 -> 33 Bus Voltage Mux/18
  V Converter Bus 19/1 -> Phase A RMS Bus 19/1
  Phase A RMS Bus 19/1 -> Per unit Bus 19/1
  Per unit Bus 19/1 -> 33 Bus Voltage Mux/19
  V Converter Bus 20/1 -> Phase A RMS Bus 20/1
  Phase A RMS Bus 20/1 -> Per unit Bus 20/1
  Per unit Bus 20/1 -> 33 Bus Voltage Mux/20
  V Converter Bus 21/1 -> Phase A RMS Bus 21/1
  Phase A RMS Bus 21/1 -> Per unit Bus 21/1
  Per unit Bus 21/1 -> 33 Bus Voltage Mux/21
  V Converter Bus 22/1 -> Phase A RMS Bus 22/1
  Phase A RMS Bus 22/1 -> Per unit Bus 22/1
  Per unit Bus 22/1 -> 33 Bus Voltage Mux/22
  V Converter Bus 23/1 -> Phase A RMS Bus 23/1
  Phase A RMS Bus 23/1 -> Per unit Bus 23/1
  Per unit Bus 23/1 -> 33 Bus Voltage Mux/23
  V Converter Bus 24/1 -> Phase A RMS Bus 24/1
  Phase A RMS Bus 24/1 -> Per unit Bus 24/1
  Per unit Bus 24/1 -> 33 Bus Voltage Mux/24
  V Converter Bus 25/1 -> Phase A RMS Bus 25/1
  Phase A RMS Bus 25/1 -> Per unit Bus 25/1
  Per unit Bus 25/1 -> 33 Bus Voltage Mux/25
  V Converter Bus 26/1 -> Phase A RMS Bus 26/1
  Phase A RMS Bus 26/1 -> Per unit Bus 26/1
  Per unit Bus 26/1 -> 33 Bus Voltage Mux/26
  V Converter Bus 27/1 -> Phase A RMS Bus 27/1
  Phase A RMS Bus 27/1 -> Per unit Bus 27/1
  Per unit Bus 27/1 -> 33 Bus Voltage Mux/27
  V Converter Bus 28/1 -> Phase A RMS Bus 28/1
  Phase A RMS Bus 28/1 -> Per unit Bus 28/1
  Per unit Bus 28/1 -> 33 Bus Voltage Mux/28
  V Converter Bus 29/1 -> Phase A RMS Bus 29/1
  Phase A RMS Bus 29/1 -> Per unit Bus 29/1
  Per unit Bus 29/1 -> 33 Bus Voltage Mux/29
  V Converter Bus 30/1 -> Phase A RMS Bus 30/1
  Phase A RMS Bus 30/1 -> Per unit Bus 30/1
  Per unit Bus 30/1 -> 33 Bus Voltage Mux/30
  V Converter Bus 31/1 -> Phase A RMS Bus 31/1
  Phase A RMS Bus 31/1 -> Per unit Bus 31/1
  Per unit Bus 31/1 -> 33 Bus Voltage Mux/31
  V Converter Bus 32/1 -> Phase A RMS Bus 32/1
  Phase A RMS Bus 32/1 -> Per unit Bus 32/1
  Per unit Bus 32/1 -> 33 Bus Voltage Mux/32
  V Converter Bus 33/1 -> Phase A RMS Bus 33/1
  Phase A RMS Bus 33/1 -> Per unit Bus 33/1
  Per unit Bus 33/1 -> 33 Bus Voltage Mux/33
  33 Bus Voltage Mux/1 -> Vbus pu/1
  Load scale/1 -> P Load Bus 02/1, Q Load Bus 02/1, P Load Bus 03/1, Q Load Bus 03/1, P Load Bus 04/1, Q Load Bus 04/1, P Load Bus 05/1, Q Load Bus 05/1, P Load Bus 06/1, Q Load Bus 06/1, P Load Bus 07/1, Q Load Bus 07/1, P Load Bus 08/1, Q Load Bus 08/1, P Load Bus 09/1, Q Load Bus 09/1, P Load Bus 10/1, Q Load Bus 10/1, P Load Bus 11/1, Q Load Bus 11/1, P Load Bus 12/1, Q Load Bus 12/1, P Load Bus 13/1, Q Load Bus 13/1, P Load Bus 14/1, Q Load Bus 14/1, P Load Bus 15/1, Q Load Bus 15/1, P Load Bus 16/1, Q Load Bus 16/1, P Load Bus 17/1, Q Load Bus 17/1, P Load Bus 18/1, Q Load Bus 18/1, P Load Bus 19/1, Q Load Bus 19/1, P Load Bus 20/1, Q Load Bus 20/1, P Load Bus 21/1, Q Load Bus 21/1, P Load Bus 22/1, Q Load Bus 22/1, P Load Bus 23/1, Q Load Bus 23/1, P Load Bus 24/1, Q Load Bus 24/1, P Load Bus 25/1, Q Load Bus 25/1, P Load Bus 26/1, Q Load Bus 26/1, P Load Bus 27/1, Q Load Bus 27/1, P Load Bus 28/1, Q Load Bus 28/1, P Load Bus 29/1, Q Load Bus 29/1, P Load Bus 30/1, Q Load Bus 30/1, P Load Bus 31/1, Q Load Bus 31/1, P Load Bus 32/1, Q Load Bus 32/1, P Load Bus 33/1, Q Load Bus 33/1
  P Load Bus 02/1 -> P PS Bus 02/1
  Q Load Bus 02/1 -> Q PS Bus 02/1
  P Load Bus 03/1 -> P PS Bus 03/1
  Q Load Bus 03/1 -> Q PS Bus 03/1
  P Load Bus 04/1 -> P PS Bus 04/1
  Q Load Bus 04/1 -> Q PS Bus 04/1
  P Load Bus 05/1 -> P PS Bus 05/1
  Q Load Bus 05/1 -> Q PS Bus 05/1
  P Load Bus 06/1 -> P PS Bus 06/1
  Q Load Bus 06/1 -> Q PS Bus 06/1
  P Load Bus 07/1 -> P PS Bus 07/1
  Q Load Bus 07/1 -> Q PS Bus 07/1
  P Load Bus 08/1 -> P PS Bus 08/1
  Q Load Bus 08/1 -> Q PS Bus 08/1
  P Load Bus 09/1 -> P PS Bus 09/1
  Q Load Bus 09/1 -> Q PS Bus 09/1
  P Load Bus 10/1 -> P PS Bus 10/1
  Q Load Bus 10/1 -> Q PS Bus 10/1
  P Load Bus 11/1 -> P PS Bus 11/1
  Q Load Bus 11/1 -> Q PS Bus 11/1
  P Load Bus 12/1 -> P PS Bus 12/1
  Q Load Bus 12/1 -> Q PS Bus 12/1
  P Load Bus 13/1 -> P PS Bus 13/1
  Q Load Bus 13/1 -> Q PS Bus 13/1
  P Load Bus 14/1 -> P PS Bus 14/1
  Q Load Bus 14/1 -> Q PS Bus 14/1
  P Load Bus 15/1 -> P PS Bus 15/1
  Q Load Bus 15/1 -> Q PS Bus 15/1
  P Load Bus 16/1 -> P PS Bus 16/1
  Q Load Bus 16/1 -> Q PS Bus 16/1
  P Load Bus 17/1 -> P PS Bus 17/1
  Q Load Bus 17/1 -> Q PS Bus 17/1
  P Load Bus 18/1 -> P PS Bus 18/1
  Q Load Bus 18/1 -> Q PS Bus 18/1
  P Load Bus 19/1 -> P PS Bus 19/1
  Q Load Bus 19/1 -> Q PS Bus 19/1
  P Load Bus 20/1 -> P PS Bus 20/1
  Q Load Bus 20/1 -> Q PS Bus 20/1
  P Load Bus 21/1 -> P PS Bus 21/1
  Q Load Bus 21/1 -> Q PS Bus 21/1
  P Load Bus 22/1 -> P PS Bus 22/1
  Q Load Bus 22/1 -> Q PS Bus 22/1
  P Load Bus 23/1 -> P PS Bus 23/1
  Q Load Bus 23/1 -> Q PS Bus 23/1
  P Load Bus 24/1 -> P PS Bus 24/1
  Q Load Bus 24/1 -> Q PS Bus 24/1
  P Load Bus 25/1 -> P PS Bus 25/1
  Q Load Bus 25/1 -> Q PS Bus 25/1
  P Load Bus 26/1 -> P PS Bus 26/1
  Q Load Bus 26/1 -> Q PS Bus 26/1
  P Load Bus 27/1 -> P PS Bus 27/1
  Q Load Bus 27/1 -> Q PS Bus 27/1
  P Load Bus 28/1 -> P PS Bus 28/1
  Q Load Bus 28/1 -> Q PS Bus 28/1
  P Load Bus 29/1 -> P PS Bus 29/1
  Q Load Bus 29/1 -> Q PS Bus 29/1
  P Load Bus 30/1 -> P PS Bus 30/1
  Q Load Bus 30/1 -> Q PS Bus 30/1
  P Load Bus 31/1 -> P PS Bus 31/1
  Q Load Bus 31/1 -> Q PS Bus 31/1
  P Load Bus 32/1 -> P PS Bus 32/1
  Q Load Bus 32/1 -> Q PS Bus 32/1
  P Load Bus 33/1 -> P PS Bus 33/1
  Q Load Bus 33/1 -> Q PS Bus 33/1
  Irradiance/1 -> Irradiance Wm2/1
  Irradiance Wm2/1 -> Irradiance PS/1
  PV P commands/1 -> P Command PV 01/1, P Command PV 02/1, P Command PV 03/1, P Command PV 04/1, P Command PV 05/1, P Command PV 06/1
  PV Q commands/1 -> Q Command PV 01/1, Q Command PV 02/1, Q Command PV 03/1, Q Command PV 04/1, Q Command PV 05/1, Q Command PV 06/1
  PV curtail commands/1 -> Curtail Command PV 01/1, Curtail Command PV 02/1, Curtail Command PV 03/1, Curtail Command PV 04/1, Curtail Command PV 05/1, Curtail Command PV 06/1
  P Command PV 01/1 -> Neg P PV 06/1, Total PV P/1
  Q Command PV 01/1 -> Neg Q PV 06/1, Total PV Q/1
  Neg P PV 06/1 -> P PV PS 06/1
  Neg Q PV 06/1 -> Q PV PS 06/1
  Curtail Command PV 01/1 -> Total Curtailment/1
  P Command PV 02/1 -> Neg P PV 14/1, Total PV P/2
  Q Command PV 02/1 -> Neg Q PV 14/1, Total PV Q/2
  Neg P PV 14/1 -> P PV PS 14/1
  Neg Q PV 14/1 -> Q PV PS 14/1
  Curtail Command PV 02/1 -> Total Curtailment/2
  P Command PV 03/1 -> Neg P PV 18/1, Total PV P/3
  Q Command PV 03/1 -> Neg Q PV 18/1, Total PV Q/3
  Neg P PV 18/1 -> P PV PS 18/1
  Neg Q PV 18/1 -> Q PV PS 18/1
  Curtail Command PV 03/1 -> Total Curtailment/3
  P Command PV 04/1 -> Neg P PV 25/1, Total PV P/4
  Q Command PV 04/1 -> Neg Q PV 25/1, Total PV Q/4
  Neg P PV 25/1 -> P PV PS 25/1
  Neg Q PV 25/1 -> Q PV PS 25/1
  Curtail Command PV 04/1 -> Total Curtailment/4
  P Command PV 05/1 -> Neg P PV 30/1, Total PV P/5
  Q Command PV 05/1 -> Neg Q PV 30/1, Total PV Q/5
  Neg P PV 30/1 -> P PV PS 30/1
  Neg Q PV 30/1 -> Q PV PS 30/1
  Curtail Command PV 05/1 -> Total Curtailment/5
  P Command PV 06/1 -> Neg P PV 33/1, Total PV P/6
  Q Command PV 06/1 -> Neg Q PV 33/1, Total PV Q/6
  Neg P PV 33/1 -> P PV PS 33/1
  Neg Q PV 33/1 -> Q PV PS 33/1
  Curtail Command PV 06/1 -> Total Curtailment/6
  Total PV P/1 -> PV P kW/1
  Total PV Q/1 -> PV Q kVAr/1
  Total Curtailment/1 -> Curtailment kW/1
  connections:
  12.66 kV Grid/LConn1 -- Electrical Reference/LConn1 -- DC MPPT Equivalent R Bus 06/RConn1 -- Solar Cell Array Bus 06/RConn1 -- DC MPPT Equivalent R Bus 14/RConn1 -- Solar Cell Array Bus 14/RConn1 -- DC MPPT Equivalent R Bus 18/RConn1 -- Solar Cell Array Bus 18/RConn1 -- DC MPPT Equivalent R Bus 25/RConn1 -- Solar Cell Array Bus 25/RConn1 -- DC MPPT Equivalent R Bus 30/RConn1 -- Solar Cell Array Bus 30/RConn1 -- DC MPPT Equivalent R Bus 33/RConn1 -- Solar Cell Array Bus 33/RConn1
  Solver Configuration/RConn1 -- Line 01-02/LConn1 -- 12.66 kV Grid/RConn1 -- V Sensor Bus 01/LConn1
  Line 02-03/LConn1 -- Line 01-02/RConn1 -- Line 02-19/LConn1 -- V Sensor Bus 02/LConn1 -- Load Bus 02/LConn1
  Line 03-04/LConn1 -- Line 02-03/RConn1 -- Line 03-23/LConn1 -- V Sensor Bus 03/LConn1 -- Load Bus 03/LConn1
  Line 04-05/LConn1 -- Line 03-04/RConn1 -- V Sensor Bus 04/LConn1 -- Load Bus 04/LConn1
  Line 05-06/LConn1 -- Line 04-05/RConn1 -- V Sensor Bus 05/LConn1 -- Load Bus 05/LConn1
  Line 06-07/LConn1 -- Line 05-06/RConn1 -- Line 06-26/LConn1 -- V Sensor Bus 06/LConn1 -- Load Bus 06/LConn1 -- Average PQ Inverter Bus 06/LConn1
  Line 07-08/LConn1 -- Line 06-07/RConn1 -- V Sensor Bus 07/LConn1 -- Load Bus 07/LConn1
  Line 08-09/LConn1 -- Line 07-08/RConn1 -- V Sensor Bus 08/LConn1 -- Load Bus 08/LConn1
  Line 09-10/LConn1 -- Line 08-09/RConn1 -- V Sensor Bus 09/LConn1 -- Load Bus 09/LConn1
  Line 10-11/LConn1 -- Line 09-10/RConn1 -- V Sensor Bus 10/LConn1 -- Load Bus 10/LConn1
  Line 11-12/LConn1 -- Line 10-11/RConn1 -- V Sensor Bus 11/LConn1 -- Load Bus 11/LConn1
  Line 12-13/LConn1 -- Line 11-12/RConn1 -- V Sensor Bus 12/LConn1 -- Load Bus 12/LConn1
  Line 13-14/LConn1 -- Line 12-13/RConn1 -- V Sensor Bus 13/LConn1 -- Load Bus 13/LConn1
  Line 14-15/LConn1 -- Line 13-14/RConn1 -- V Sensor Bus 14/LConn1 -- Load Bus 14/LConn1 -- Average PQ Inverter Bus 14/LConn1
  Line 15-16/LConn1 -- Line 14-15/RConn1 -- V Sensor Bus 15/LConn1 -- Load Bus 15/LConn1
  Line 16-17/LConn1 -- Line 15-16/RConn1 -- V Sensor Bus 16/LConn1 -- Load Bus 16/LConn1
  Line 17-18/LConn1 -- Line 16-17/RConn1 -- V Sensor Bus 17/LConn1 -- Load Bus 17/LConn1
  Line 19-20/LConn1 -- Line 02-19/RConn1 -- V Sensor Bus 19/LConn1 -- Load Bus 19/LConn1
  Line 20-21/LConn1 -- Line 19-20/RConn1 -- V Sensor Bus 20/LConn1 -- Load Bus 20/LConn1
  Line 21-22/LConn1 -- Line 20-21/RConn1 -- V Sensor Bus 21/LConn1 -- Load Bus 21/LConn1
  Line 23-24/LConn1 -- Line 03-23/RConn1 -- V Sensor Bus 23/LConn1 -- Load Bus 23/LConn1
  Line 24-25/LConn1 -- Line 23-24/RConn1 -- V Sensor Bus 24/LConn1 -- Load Bus 24/LConn1
  Line 26-27/LConn1 -- Line 06-26/RConn1 -- V Sensor Bus 26/LConn1 -- Load Bus 26/LConn1
  Line 27-28/LConn1 -- Line 26-27/RConn1 -- V Sensor Bus 27/LConn1 -- Load Bus 27/LConn1
  Line 28-29/LConn1 -- Line 27-28/RConn1 -- V Sensor Bus 28/LConn1 -- Load Bus 28/LConn1
  Line 29-30/LConn1 -- Line 28-29/RConn1 -- V Sensor Bus 29/LConn1 -- Load Bus 29/LConn1
  Line 30-31/LConn1 -- Line 29-30/RConn1 -- V Sensor Bus 30/LConn1 -- Load Bus 30/LConn1 -- Average PQ Inverter Bus 30/LConn1
  Line 31-32/LConn1 -- Line 30-31/RConn1 -- V Sensor Bus 31/LConn1 -- Load Bus 31/LConn1
  Line 32-33/LConn1 -- Line 31-32/RConn1 -- V Sensor Bus 32/LConn1 -- Load Bus 32/LConn1
  V Sensor Bus 01/RConn1 -- RMS Bus 01/LConn1
  RMS Bus 01/RConn1 -- V Converter Bus 01/LConn1
  V Sensor Bus 02/RConn1 -- RMS Bus 02/LConn1
  RMS Bus 02/RConn1 -- V Converter Bus 02/LConn1
  V Sensor Bus 03/RConn1 -- RMS Bus 03/LConn1
  RMS Bus 03/RConn1 -- V Converter Bus 03/LConn1
  V Sensor Bus 04/RConn1 -- RMS Bus 04/LConn1
  RMS Bus 04/RConn1 -- V Converter Bus 04/LConn1
  V Sensor Bus 05/RConn1 -- RMS Bus 05/LConn1
  RMS Bus 05/RConn1 -- V Converter Bus 05/LConn1
  V Sensor Bus 06/RConn1 -- RMS Bus 06/LConn1
  RMS Bus 06/RConn1 -- V Converter Bus 06/LConn1
  V Sensor Bus 07/RConn1 -- RMS Bus 07/LConn1
  RMS Bus 07/RConn1 -- V Converter Bus 07/LConn1
  V Sensor Bus 08/RConn1 -- RMS Bus 08/LConn1
  RMS Bus 08/RConn1 -- V Converter Bus 08/LConn1
  V Sensor Bus 09/RConn1 -- RMS Bus 09/LConn1
  RMS Bus 09/RConn1 -- V Converter Bus 09/LConn1
  V Sensor Bus 10/RConn1 -- RMS Bus 10/LConn1
  RMS Bus 10/RConn1 -- V Converter Bus 10/LConn1
  V Sensor Bus 11/RConn1 -- RMS Bus 11/LConn1
  RMS Bus 11/RConn1 -- V Converter Bus 11/LConn1
  V Sensor Bus 12/RConn1 -- RMS Bus 12/LConn1
  RMS Bus 12/RConn1 -- V Converter Bus 12/LConn1
  V Sensor Bus 13/RConn1 -- RMS Bus 13/LConn1
  RMS Bus 13/RConn1 -- V Converter Bus 13/LConn1
  V Sensor Bus 14/RConn1 -- RMS Bus 14/LConn1
  RMS Bus 14/RConn1 -- V Converter Bus 14/LConn1
  V Sensor Bus 15/RConn1 -- RMS Bus 15/LConn1
  RMS Bus 15/RConn1 -- V Converter Bus 15/LConn1
  V Sensor Bus 16/RConn1 -- RMS Bus 16/LConn1
  RMS Bus 16/RConn1 -- V Converter Bus 16/LConn1
  V Sensor Bus 17/RConn1 -- RMS Bus 17/LConn1
  RMS Bus 17/RConn1 -- V Converter Bus 17/LConn1
  V Sensor Bus 18/LConn1 -- Line 17-18/RConn1 -- Load Bus 18/LConn1 -- Average PQ Inverter Bus 18/LConn1
  V Sensor Bus 18/RConn1 -- RMS Bus 18/LConn1
  RMS Bus 18/RConn1 -- V Converter Bus 18/LConn1
  V Sensor Bus 19/RConn1 -- RMS Bus 19/LConn1
  RMS Bus 19/RConn1 -- V Converter Bus 19/LConn1
  V Sensor Bus 20/RConn1 -- RMS Bus 20/LConn1
  RMS Bus 20/RConn1 -- V Converter Bus 20/LConn1
  V Sensor Bus 21/RConn1 -- RMS Bus 21/LConn1
  RMS Bus 21/RConn1 -- V Converter Bus 21/LConn1
  V Sensor Bus 22/LConn1 -- Line 21-22/RConn1 -- Load Bus 22/LConn1
  V Sensor Bus 22/RConn1 -- RMS Bus 22/LConn1
  RMS Bus 22/RConn1 -- V Converter Bus 22/LConn1
  V Sensor Bus 23/RConn1 -- RMS Bus 23/LConn1
  RMS Bus 23/RConn1 -- V Converter Bus 23/LConn1
  V Sensor Bus 24/RConn1 -- RMS Bus 24/LConn1
  RMS Bus 24/RConn1 -- V Converter Bus 24/LConn1
  V Sensor Bus 25/LConn1 -- Line 24-25/RConn1 -- Load Bus 25/LConn1 -- Average PQ Inverter Bus 25/LConn1
  V Sensor Bus 25/RConn1 -- RMS Bus 25/LConn1
  RMS Bus 25/RConn1 -- V Converter Bus 25/LConn1
  V Sensor Bus 26/RConn1 -- RMS Bus 26/LConn1
  RMS Bus 26/RConn1 -- V Converter Bus 26/LConn1
  V Sensor Bus 27/RConn1 -- RMS Bus 27/LConn1
  RMS Bus 27/RConn1 -- V Converter Bus 27/LConn1
  V Sensor Bus 28/RConn1 -- RMS Bus 28/LConn1
  RMS Bus 28/RConn1 -- V Converter Bus 28/LConn1
  V Sensor Bus 29/RConn1 -- RMS Bus 29/LConn1
  RMS Bus 29/RConn1 -- V Converter Bus 29/LConn1
  V Sensor Bus 30/RConn1 -- RMS Bus 30/LConn1
  RMS Bus 30/RConn1 -- V Converter Bus 30/LConn1
  V Sensor Bus 31/RConn1 -- RMS Bus 31/LConn1
  RMS Bus 31/RConn1 -- V Converter Bus 31/LConn1
  V Sensor Bus 32/RConn1 -- RMS Bus 32/LConn1
  RMS Bus 32/RConn1 -- V Converter Bus 32/LConn1
  V Sensor Bus 33/LConn1 -- Line 32-33/RConn1 -- Load Bus 33/LConn1 -- Average PQ Inverter Bus 33/LConn1
  V Sensor Bus 33/RConn1 -- RMS Bus 33/LConn1
  RMS Bus 33/RConn1 -- V Converter Bus 33/LConn1
  P PS Bus 02/RConn1 -- Load Bus 02/LConn2
  Q PS Bus 02/RConn1 -- Load Bus 02/LConn3
  P PS Bus 03/RConn1 -- Load Bus 03/LConn2
  Q PS Bus 03/RConn1 -- Load Bus 03/LConn3
  P PS Bus 04/RConn1 -- Load Bus 04/LConn2
  Q PS Bus 04/RConn1 -- Load Bus 04/LConn3
  P PS Bus 05/RConn1 -- Load Bus 05/LConn2
  Q PS Bus 05/RConn1 -- Load Bus 05/LConn3
  P PS Bus 06/RConn1 -- Load Bus 06/LConn2
  Q PS Bus 06/RConn1 -- Load Bus 06/LConn3
  P PS Bus 07/RConn1 -- Load Bus 07/LConn2
  Q PS Bus 07/RConn1 -- Load Bus 07/LConn3
  P PS Bus 08/RConn1 -- Load Bus 08/LConn2
  Q PS Bus 08/RConn1 -- Load Bus 08/LConn3
  P PS Bus 09/RConn1 -- Load Bus 09/LConn2
  Q PS Bus 09/RConn1 -- Load Bus 09/LConn3
  P PS Bus 10/RConn1 -- Load Bus 10/LConn2
  Q PS Bus 10/RConn1 -- Load Bus 10/LConn3
  P PS Bus 11/RConn1 -- Load Bus 11/LConn2
  Q PS Bus 11/RConn1 -- Load Bus 11/LConn3
  P PS Bus 12/RConn1 -- Load Bus 12/LConn2
  Q PS Bus 12/RConn1 -- Load Bus 12/LConn3
  P PS Bus 13/RConn1 -- Load Bus 13/LConn2
  Q PS Bus 13/RConn1 -- Load Bus 13/LConn3
  P PS Bus 14/RConn1 -- Load Bus 14/LConn2
  Q PS Bus 14/RConn1 -- Load Bus 14/LConn3
  P PS Bus 15/RConn1 -- Load Bus 15/LConn2
  Q PS Bus 15/RConn1 -- Load Bus 15/LConn3
  P PS Bus 16/RConn1 -- Load Bus 16/LConn2
  Q PS Bus 16/RConn1 -- Load Bus 16/LConn3
  P PS Bus 17/RConn1 -- Load Bus 17/LConn2
  Q PS Bus 17/RConn1 -- Load Bus 17/LConn3
  P PS Bus 18/RConn1 -- Load Bus 18/LConn2
  Q PS Bus 18/RConn1 -- Load Bus 18/LConn3
  P PS Bus 19/RConn1 -- Load Bus 19/LConn2
  Q PS Bus 19/RConn1 -- Load Bus 19/LConn3
  P PS Bus 20/RConn1 -- Load Bus 20/LConn2
  Q PS Bus 20/RConn1 -- Load Bus 20/LConn3
  P PS Bus 21/RConn1 -- Load Bus 21/LConn2
  Q PS Bus 21/RConn1 -- Load Bus 21/LConn3
  P PS Bus 22/RConn1 -- Load Bus 22/LConn2
  Q PS Bus 22/RConn1 -- Load Bus 22/LConn3
  P PS Bus 23/RConn1 -- Load Bus 23/LConn2
  Q PS Bus 23/RConn1 -- Load Bus 23/LConn3
  P PS Bus 24/RConn1 -- Load Bus 24/LConn2
  Q PS Bus 24/RConn1 -- Load Bus 24/LConn3
  P PS Bus 25/RConn1 -- Load Bus 25/LConn2
  Q PS Bus 25/RConn1 -- Load Bus 25/LConn3
  P PS Bus 26/RConn1 -- Load Bus 26/LConn2
  Q PS Bus 26/RConn1 -- Load Bus 26/LConn3
  P PS Bus 27/RConn1 -- Load Bus 27/LConn2
  Q PS Bus 27/RConn1 -- Load Bus 27/LConn3
  P PS Bus 28/RConn1 -- Load Bus 28/LConn2
  Q PS Bus 28/RConn1 -- Load Bus 28/LConn3
  P PS Bus 29/RConn1 -- Load Bus 29/LConn2
  Q PS Bus 29/RConn1 -- Load Bus 29/LConn3
  P PS Bus 30/RConn1 -- Load Bus 30/LConn2
  Q PS Bus 30/RConn1 -- Load Bus 30/LConn3
  P PS Bus 31/RConn1 -- Load Bus 31/LConn2
  Q PS Bus 31/RConn1 -- Load Bus 31/LConn3
  P PS Bus 32/RConn1 -- Load Bus 32/LConn2
  Q PS Bus 32/RConn1 -- Load Bus 32/LConn3
  P PS Bus 33/RConn1 -- Load Bus 33/LConn2
  Q PS Bus 33/RConn1 -- Load Bus 33/LConn3
  P PV PS 06/RConn1 -- Average PQ Inverter Bus 06/LConn2
  Q PV PS 06/RConn1 -- Average PQ Inverter Bus 06/LConn3
  Solar Cell Array Bus 06/LConn1 -- Irradiance PS/RConn1 -- Solar Cell Array Bus 14/LConn1 -- Solar Cell Array Bus 18/LConn1 -- Solar Cell Array Bus 25/LConn1 -- Solar Cell Array Bus 30/LConn1 -- Solar Cell Array Bus 33/LConn1
  Solar Cell Array Bus 06/LConn2 -- DC MPPT Equivalent R Bus 06/LConn1
  P PV PS 14/RConn1 -- Average PQ Inverter Bus 14/LConn2
  Q PV PS 14/RConn1 -- Average PQ Inverter Bus 14/LConn3
  Solar Cell Array Bus 14/LConn2 -- DC MPPT Equivalent R Bus 14/LConn1
  P PV PS 18/RConn1 -- Average PQ Inverter Bus 18/LConn2
  Q PV PS 18/RConn1 -- Average PQ Inverter Bus 18/LConn3
  Solar Cell Array Bus 18/LConn2 -- DC MPPT Equivalent R Bus 18/LConn1
  P PV PS 25/RConn1 -- Average PQ Inverter Bus 25/LConn2
  Q PV PS 25/RConn1 -- Average PQ Inverter Bus 25/LConn3
  Solar Cell Array Bus 25/LConn2 -- DC MPPT Equivalent R Bus 25/LConn1
  P PV PS 30/RConn1 -- Average PQ Inverter Bus 30/LConn2
  Q PV PS 30/RConn1 -- Average PQ Inverter Bus 30/LConn3
  Solar Cell Array Bus 30/LConn2 -- DC MPPT Equivalent R Bus 30/LConn1
  P PV PS 33/RConn1 -- Average PQ Inverter Bus 33/LConn2
  Q PV PS 33/RConn1 -- Average PQ Inverter Bus 33/LConn3
  Solar Cell Array Bus 33/LConn2 -- DC MPPT Equivalent R Bus 33/LConn1
